simulink model "L4Zadatak2b"  (Simulink 8.9)
settings: Solver=ode45  StartTime=0.0  StopTime=100  RelTol=1e-3  EnableMultiTasking=on
settings Model: Creator=student  LastModifiedBy=korisnik
settings OptimizationCC: ExpressionDepthLimit=2147483647
settings DebuggingCC: SolverPrmCheckMsg=warning

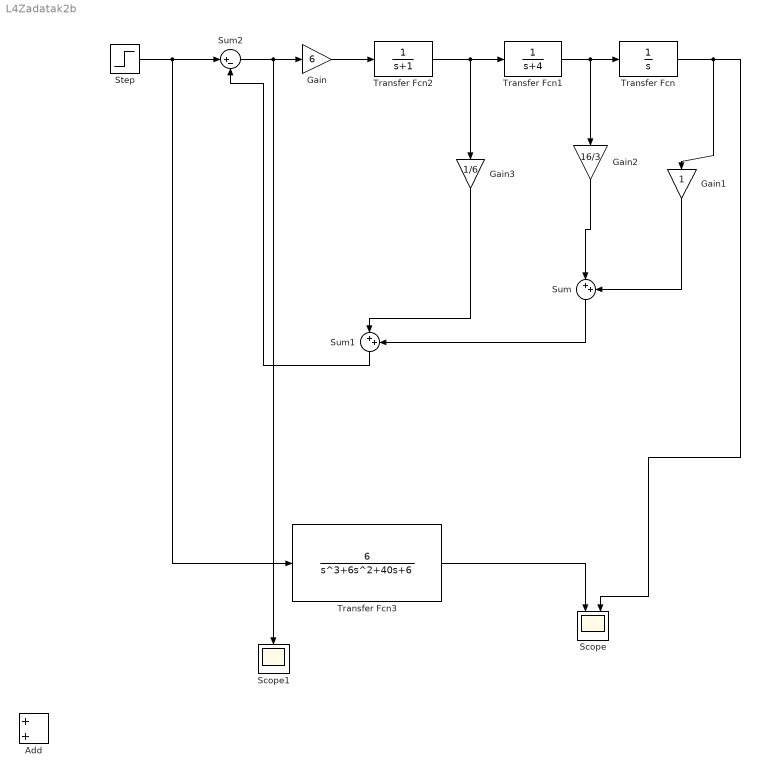
== system L4Zadatak2b ==
  Add : Sum
  Gain : Gain  Gain=6
  Gain1 : Gain
  Gain2 : Gain  Gain=16/3
  Gain3 : Gain  Gain=1/6
  Scope : Scope  NumInputPorts=2
  Scope1 : Scope
  Step : Step  SampleTime=0
  Sum : Sum  Inputs=|++
  Sum1 : Sum  Inputs=|++
  Sum2 : Sum  Inputs=|+-
  Transfer Fcn : TransferFcn  Denominator=[1 0]
  Transfer Fcn1 : TransferFcn  Denominator=[1 4]
  Transfer Fcn2 : TransferFcn  Denominator=[1 1]
  Transfer Fcn3 : TransferFcn  Numerator=[6]  Denominator=[1 6 40 6]
  wires:
  Gain/1 -> Transfer Fcn2/1
  Transfer Fcn2/1 -> Transfer Fcn1/1, Gain3/1
  Transfer Fcn1/1 -> Gain2/1, Transfer Fcn/1
  Transfer Fcn/1 -> Gain1/1, Scope/2
  Gain1/1 -> Sum/2
  Gain2/1 -> Sum/1
  Gain3/1 -> Sum1/1
  Sum/1 -> Sum1/2
  Sum1/1 -> Sum2/2
  Step/1 -> Sum2/1, Transfer Fcn3/1
  Sum2/1 -> Gain/1, Scope1/1
  Transfer Fcn3/1 -> Scope/1
